simulink model "part2"  (R2014a)
settings: Solver=ode45  StartTime=0.0  StopTime=10.0  RelTol=1e-3
settings Model: Creator=SuperUser  LastModifiedBy=SuperUser

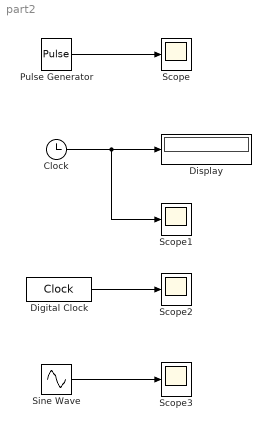
== system part2 ==
  Clock : Clock
      settings: Decimation=20
  Digital Clock : DigitalClock
  Display : Display
  Pulse Generator : DiscretePulseGenerator  PulseType=Time based  Period=5  PulseWidth=50
  Scope{,1..3} (4 alike) : Scope
      Scope1 settings: YMin=0  YMax=20
      Scope2 settings: SaveName=ScopeData2
      Scope3 settings: SaveName=ScopeData3
  Sine Wave : Sin  SampleTime=0
  wires:
  Pulse Generator/1 -> Scope/1
  Clock/1 -> Display/1, Scope1/1
  Digital Clock/1 -> Scope2/1
  Sine Wave/1 -> Scope3/1
